simulink model "Asynchronous_motor"  (R2024a)
settings: Solver=VariableStepAuto  StartTime=0.0  StopTime=10.0  RelTol=1e-3
values from neighbouring files (symbols this model uses):
  B = 0    [setting.m]
  f_rated = 50    [setting.m]
  Ids_rated = V_max / sqrt(Rs^2 + (w_rated * Ls)^2)    [setting.m]
  J = 0.0252    [setting.m]
  Kac = 1 / Kpc    (= 0.063680128597)    [setting.m]
  Kas = 1 / Kps    [setting.m]
  Kic = R * wcc    (= 2896.1527295)    [setting.m]
  Kis = Kps * wcs / 5    [setting.m]
  Kpc = L * wcc    (= 15.7034858759)    [setting.m]
  Kps = J * wcs / Kt    [setting.m]
  Kt = 1.5 * np * Lm^2 * Ids_rated / Lr    [setting.m]
  Llr = 1.794e-3    (= 0.001794)    [setting.m]
  Lls = 1.794e-3    (= 0.001794)    [setting.m]
  np = 2    [setting.m]
  P_rated = 3700    [setting.m]
  pxyz = sqrt(3) *Tsw / Vdc    [setting.m]
  Rr = 0.379    [setting.m]
  Rs = 0.295    [setting.m]
  Te_rated = np * P_rated / (w_syn * (1 - s_rated))    (= 48.4005443375)    [setting.m]
  Tsw = 1 / fsw    (= 0.0001)    [setting.m]
  V_max = sqrt(2) / sqrt(3) * V_rated    [setting.m]
  V_rated = 220    [setting.m]
  Vdc = 500    [setting.m]
libraries: simulink x4, spsAsynchronousMachineSIUnitsLib x1, spsDCVoltageSourceLib x1, eeTransforms x1, spsUniversalBridgeLib x1, spsabctodq0Lib x1
settings Model: Creator=d  LastModifiedBy=d

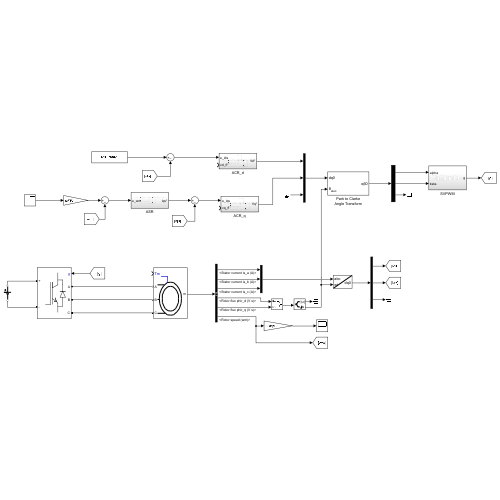
[thumbnail: Simulink's stored preview of the top-level diagram]
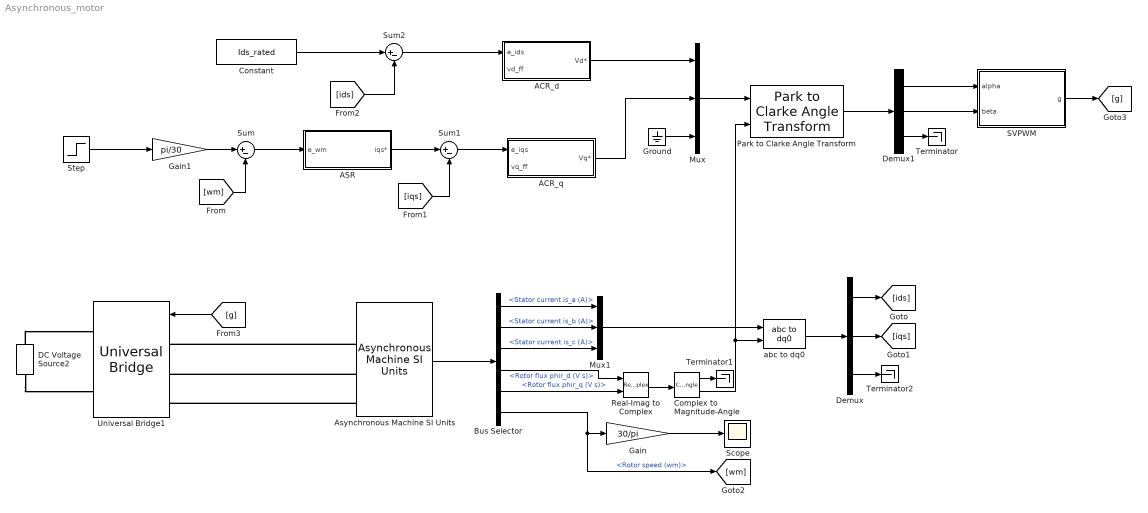
== system Asynchronous_motor ==
  ACR_d : Subsystem
  ACR_q : Subsystem
  ASR : Subsystem
  Asynchronous Machine SI Units : spsAsynchronousMachineSIUnitsLib/Asynchronous Machine SI Units  RotorType=Squirrel-cage  PresetModel=No  MechanicalLoad=Torque Tm  ShowDetailedParameters=on  ReferenceFrame=Stationary  Units=SI  MeasurementBus=off  NominalParameters=[P_rated V_rated f_rated]  VoltageRatio=1  Stator=[Rs Lls]  Rotor=[Rr Llr]  Cage1=[0.4155 0.002066]  Cage2=[0.4168 0.0003495]  Lm=Lm  Mechanical=[J B np]  PolePairs=2  InitialConditions=[1 0 0 0 0 0 0 0]  SimulateSaturation=off  Saturation=[14.03593122, 27.81365428, 53.79336849, 72.68890987, 97.98006896, 148.6815601, 215.7428561, 302.9841135, 428.7778367 ; 230, 322, 414, 460, 506, 552, 598, 644, 690]  LoadFlowParameters=1492000  TsPowergui=0  TsBlock=-1  IterativeModel=Trapezoidal non iterative  IterativeDiscreteModel=Trapezoidal non iterative  Pmec=1.492e+006
  Bus Selector : BusSelector  OutputSignals=Stator measurements.Stator current is_a (A),Stator measurements.Stator current is_b (A),Stator measurements.Stator current is_c (A),Rotor measurements.Rotor flux phir_d (V s),Rotor measurements.Rotor flux phir_q (V s),Mechanical.Rotor speed (wm)
  Complex to Magnitude-Angle : ComplexToMagnitudeAngle
  Constant : Constant  Value=Ids_rated
  DC Voltage Source2 : spsDCVoltageSourceLib/DC Voltage Source  Amplitude=Vdc  Measurements=None
  Demux : Demux  Outputs=3
  Demux1 : Demux  Outputs=3
  Gain : Gain  Gain=30/pi
  Gain1 : Gain  Gain=pi/30
  Ground : Ground
  Mux : Mux  Inputs=3
  Mux1 : Mux  Inputs=3
  Park to Clarke Angle Transform : eeTransforms/Park to Clarke Angle Transform  AxisAlignment=Q-axis
      settings: LibrarySourceBlock=|
      | ee_sl_lib/Mathematical
      | Transforms/Park to Clarke
      | Angle Transform
  Real-Imag to Complex : RealImagToComplex
  SVPWM : Subsystem
  Scope : Scope
  Step : Step  Time=0.4  Before=500  After=1400  SampleTime=0
  Sum : Sum  Inputs=|+-
  Sum1 : Sum  Inputs=|+-
  Sum2 : Sum  Inputs=|+-
  Terminator : Terminator
  Terminator1 : Terminator
  Terminator2 : Terminator
  Universal Bridge1 : spsUniversalBridgeLib/Universal Bridge  Arms=3  SnubberResistance=1e5  SnubberCapacitance=inf  Device=IGBT / Diodes  Ron=1e-3  Lon=0  ForwardVoltages="[  0  0  ]"  ForwardVoltage=0  GTOparameters=[ 10e-6 , 20e-6 ]  IGBTparameters=[ 1e-6 , 2e-6 ]  Measurements=None  Measurements_2=None  converterType=Rectifier
  abc to dq0 : spsabctodq0Lib/abc to dq0  Alignment=90 degrees behind phase A axis
  wires:
  Asynchronous Machine SI Units/1 -> Bus Selector/1
  Bus Selector/2 -> Mux1/2  "<Stator current is_b (A)>"
  Bus Selector/3 -> Mux1/3  "<Stator current is_c (A)>"
  Bus Selector/1 -> Mux1/1  "<Stator current is_a (A)>"
  Mux1/1 -> abc to dq0/1
  Complex to Magnitude-Angle/2 -> Park to Clarke Angle Transform/2, abc to dq0/2
  Bus Selector/5 -> Real-Imag to Complex/2  "<Rotor flux phir_q (V s)>"
  Bus Selector/6 -> [wm], Gain/1  "<Rotor speed (wm)>"
  Bus Selector/4 -> Real-Imag to Complex/1  "<Rotor flux phir_d (V s)>"
  Real-Imag to Complex/1 -> Complex to Magnitude-Angle/1
  Complex to Magnitude-Angle/1 -> Terminator1/1
  abc to dq0/1 -> Demux/1
  Demux/3 -> Terminator2/1
  Demux/1 -> [ids]
  Demux/2 -> [iqs]
  Gain/1 -> Scope/1
  Step/1 -> Gain1/1
  Gain1/1 -> Sum/1
  [wm] -> Sum/2
  Sum/1 -> ASR/1(e_wm)
  ASR/1(iqs*) -> Sum1/1
  [iqs] -> Sum1/2
  Sum1/1 -> ACR_q/1(e_iqs)
  Constant/1 -> Sum2/1
  [ids] -> Sum2/2
  Sum2/1 -> ACR_d/1(e_ids)
  ACR_d/1(Vd*) -> Mux/1
  ACR_q/1(Vq*) -> Mux/2
  Mux/1 -> Park to Clarke Angle Transform/1
  Ground/1 -> Mux/3
  Park to Clarke Angle Transform/1 -> Demux1/1
  Demux1/3 -> Terminator/1
  Demux1/1 -> SVPWM/1(alpha)
  Demux1/2 -> SVPWM/2(beta)
  SVPWM/1(g) -> [g]
  [g] -> Universal Bridge1/1
  connections:
  DC Voltage Source2/RConn1 -- Universal Bridge1/RConn1
  DC Voltage Source2/LConn1 -- Universal Bridge1/RConn2
  Asynchronous Machine SI Units/LConn1 -- Universal Bridge1/LConn1
  Asynchronous Machine SI Units/LConn2 -- Universal Bridge1/LConn2
  Asynchronous Machine SI Units/LConn3 -- Universal Bridge1/LConn3

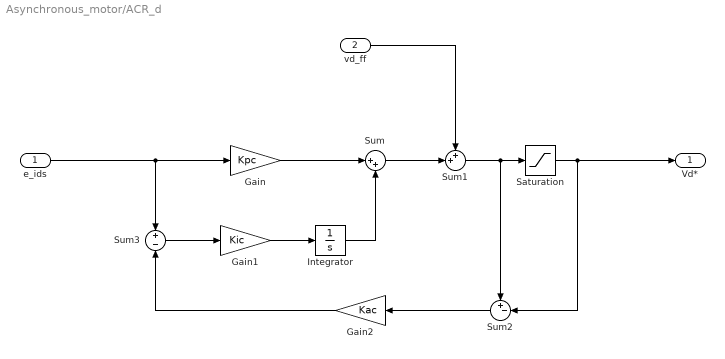
== system Asynchronous_motor/ACR_d ==
  e_ids : Inport
  vd_ff : Inport  Port=2
  Gain : Gain  Gain=Kpc
  Gain1 : Gain  Gain=Kic
  Gain2 : Gain  Gain=Kac
  Integrator : Integrator
  Saturation : Saturate  UpperLimit=V_max * 2  LowerLimit=-V_max * 2
  Sum : Sum  Inputs=|++
  Sum1 : Sum  Inputs=++|
  Sum2 : Sum  Inputs=+-|
  Sum3 : Sum  Inputs=+|-
  Vd* : Outport
  wires:
  e_ids/1 -> Sum3/1, Gain/1
  Gain1/1 -> Integrator/1
  Gain/1 -> Sum/1
  Integrator/1 -> Sum/2
  Sum/1 -> Sum1/2
  vd_ff/1 -> Sum1/1
  Sum1/1 -> Saturation/1, Sum2/1
  Saturation/1 -> Sum2/2, Vd*/1
  Sum2/1 -> Gain2/1
  Sum3/1 -> Gain1/1
  Gain2/1 -> Sum3/2

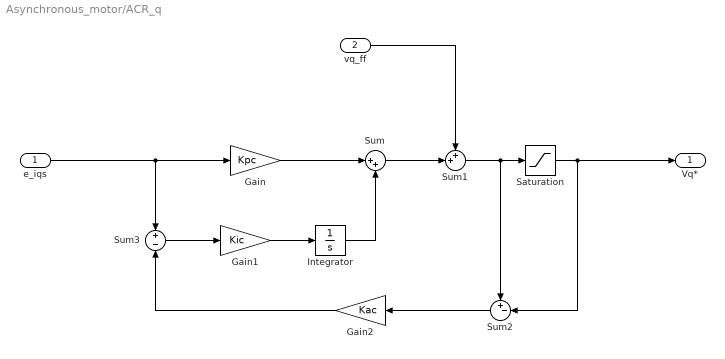
== system Asynchronous_motor/ACR_q ==
  e_iqs : Inport
  vq_ff : Inport  Port=2
  Gain : Gain  Gain=Kpc
  Gain1 : Gain  Gain=Kic
  Gain2 : Gain  Gain=Kac
  Integrator : Integrator
  Saturation : Saturate  UpperLimit=V_max * 2  LowerLimit=-V_max * 2
  Sum : Sum  Inputs=|++
  Sum1 : Sum  Inputs=++|
  Sum2 : Sum  Inputs=+-|
  Sum3 : Sum  Inputs=+|-
  Vq* : Outport
  wires:
  e_iqs/1 -> Sum3/1, Gain/1
  Gain1/1 -> Integrator/1
  Gain/1 -> Sum/1
  Integrator/1 -> Sum/2
  Sum/1 -> Sum1/2
  vq_ff/1 -> Sum1/1
  Sum1/1 -> Saturation/1, Sum2/1
  Saturation/1 -> Sum2/2, Vq*/1
  Sum2/1 -> Gain2/1
  Sum3/1 -> Gain1/1
  Gain2/1 -> Sum3/2

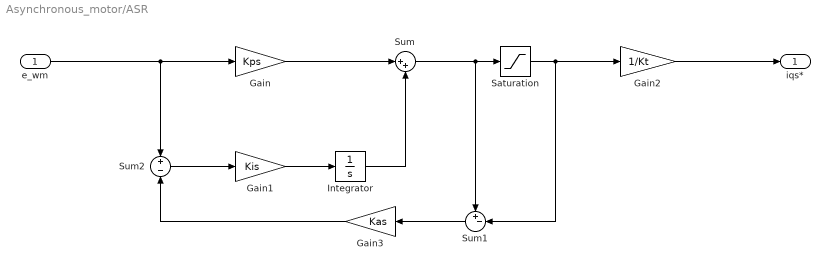
== system Asynchronous_motor/ASR ==
  e_wm : Inport
  Gain : Gain  Gain=Kps
  Gain1 : Gain  Gain=Kis
  Gain2 : Gain  Gain=1/Kt
  Gain3 : Gain  Gain=Kas
  Integrator : Integrator
  Saturation : Saturate  UpperLimit=Te_rated  LowerLimit=-Te_rated
  Sum : Sum  Inputs=|++
  Sum1 : Sum  Inputs=+-|
  Sum2 : Sum  Inputs=+|-
  iqs* : Outport
  wires:
  e_wm/1 -> Sum2/1, Gain/1
  Gain1/1 -> Integrator/1
  Gain/1 -> Sum/1
  Integrator/1 -> Sum/2
  Sum/1 -> Sum1/1, Saturation/1
  Saturation/1 -> Sum1/2, Gain2/1
  Gain2/1 -> iqs*/1
  Sum1/1 -> Gain3/1
  Sum2/1 -> Gain1/1
  Gain3/1 -> Sum2/2

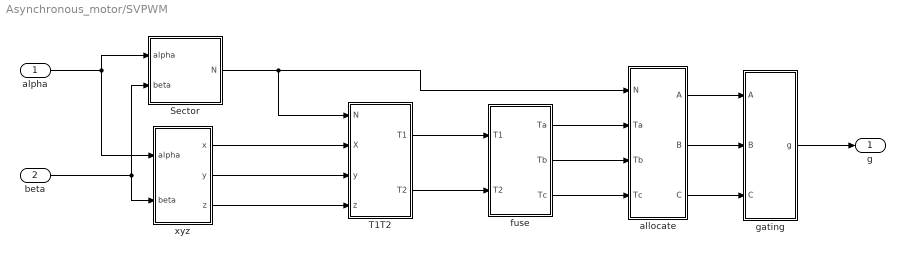
== system Asynchronous_motor/SVPWM ==
  alpha : Inport
  beta : Inport  Port=2
  Sector : Subsystem
  T1T2 : Subsystem
  allocate : Subsystem
  fuse : Subsystem
  gating : Subsystem
  xyz : Subsystem
  g : Outport
  wires:
  allocate/3(C) -> gating/3(C)
  fuse/2(Tb) -> allocate/3(Tb)
  allocate/1(A) -> gating/1(A)
  allocate/2(B) -> gating/2(B)
  xyz/2(y) -> T1T2/3(y)
  T1T2/1(T1) -> fuse/1(T1)
  xyz/3(z) -> T1T2/4(z)
  T1T2/2(T2) -> fuse/2(T2)
  fuse/3(Tc) -> allocate/4(Tc)
  Sector/1(N) -> T1T2/1(N), allocate/1(N)
  fuse/1(Ta) -> allocate/2(Ta)
  xyz/1(x) -> T1T2/2(X)
  alpha/1 -> Sector/1(alpha), xyz/1(alpha)
  beta/1 -> Sector/2(beta), xyz/2(beta)
  gating/1(g) -> g/1

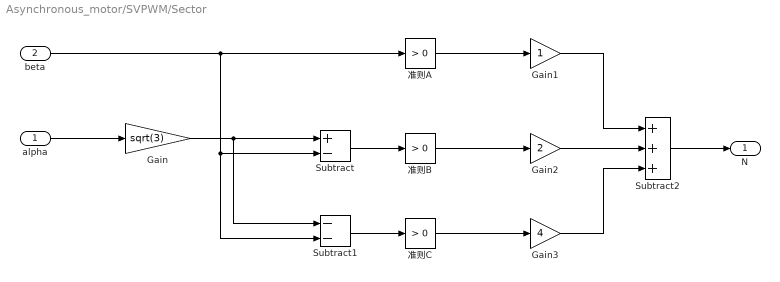
== system Asynchronous_motor/SVPWM/Sector ==
  alpha : Inport
  beta : Inport  Port=2
  Gain : Gain  Gain=sqrt(3)
  Gain1 : Gain
  Gain2 : Gain  Gain=2
  Gain3 : Gain  Gain=4
  Subtract : Sum  Inputs=+-
  Subtract1 : Sum  Inputs=--
  Subtract2 : Sum  Inputs=+++
  准则A : simulink/Logic and Bit Operations/Compare To Constant  relop=>  const=0  OutDataTypeStr=boolean
  准则B : simulink/Logic and Bit Operations/Compare To Constant  relop=>  const=0  OutDataTypeStr=boolean
  准则C : simulink/Logic and Bit Operations/Compare To Constant  relop=>  const=0  OutDataTypeStr=boolean
  N : Outport
  wires:
  beta/1 -> Subtract1/2, Subtract/2, 准则A/1
  alpha/1 -> Gain/1
  Gain/1 -> Subtract1/1, Subtract/1
  Subtract/1 -> 准则B/1
  Subtract1/1 -> 准则C/1
  准则C/1 -> Gain3/1
  准则B/1 -> Gain2/1
  准则A/1 -> Gain1/1
  Gain1/1 -> Subtract2/1
  Gain2/1 -> Subtract2/2
  Gain3/1 -> Subtract2/3
  Subtract2/1 -> N/1

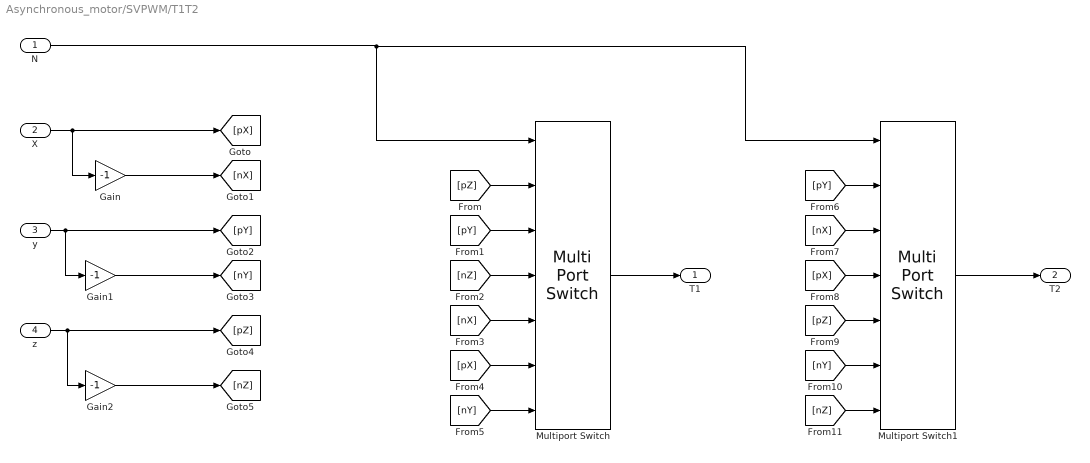
== system Asynchronous_motor/SVPWM/T1T2 ==
  N : Inport
  X : Inport  Port=2
  y : Inport  Port=3
  z : Inport  Port=4
  Gain : Gain  Gain=-1
  Gain1 : Gain  Gain=-1
  Gain2 : Gain  Gain=-1
  Multiport Switch : MultiPortSwitch  Inputs=6  SaturateOnIntegerOverflow=off  InputSameDT=off
  Multiport Switch1 : MultiPortSwitch  Inputs=6  SaturateOnIntegerOverflow=off  InputSameDT=off
  T1 : Outport
  T2 : Outport  Port=2
  wires:
  X/1 -> [pX], Gain/1
  y/1 -> [pY], Gain1/1
  z/1 -> Gain2/1, [pZ]
  Gain/1 -> [nX]
  Gain1/1 -> [nY]
  Gain2/1 -> [nZ]
  Multiport Switch/1 -> T1/1
  Multiport Switch1/1 -> T2/1
  N/1 -> Multiport Switch1/1, Multiport Switch/1
  [pZ] -> Multiport Switch/2
  [pY] -> Multiport Switch/3
  [nZ] -> Multiport Switch/4
  [nX] -> Multiport Switch/5
  [pX] -> Multiport Switch/6
  [nY] -> Multiport Switch/7
  [pY] -> Multiport Switch1/2
  [nX] -> Multiport Switch1/3
  [pX] -> Multiport Switch1/4
  [pZ] -> Multiport Switch1/5
  [nY] -> Multiport Switch1/6
  [nZ] -> Multiport Switch1/7

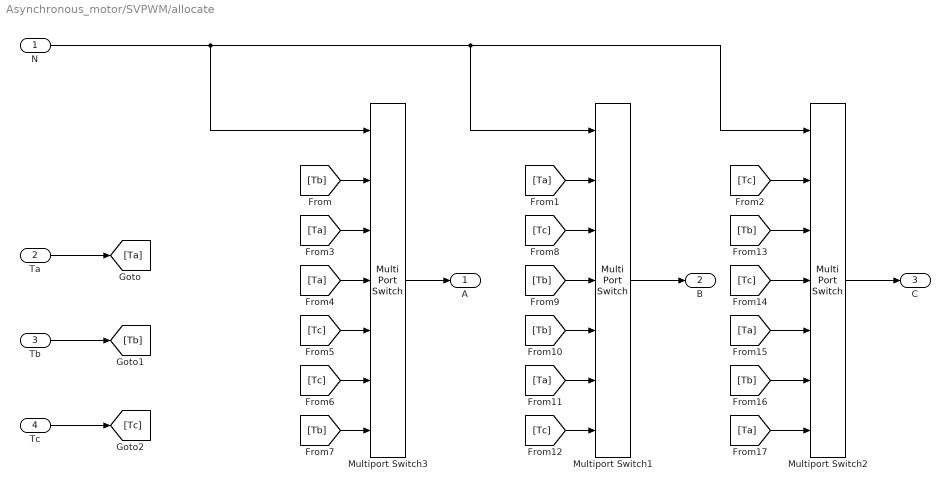
== system Asynchronous_motor/SVPWM/allocate ==
  N : Inport
  Ta : Inport  Port=2
  Tb : Inport  Port=3
  Tc : Inport  Port=4
  Multiport Switch1 : MultiPortSwitch  Inputs=6  SaturateOnIntegerOverflow=off  InputSameDT=off
  Multiport Switch2 : MultiPortSwitch  Inputs=6  SaturateOnIntegerOverflow=off  InputSameDT=off
  Multiport Switch3 : MultiPortSwitch  Inputs=6  SaturateOnIntegerOverflow=off  InputSameDT=off
  A : Outport
  B : Outport  Port=2
  C : Outport  Port=3
  wires:
  Tc/1 -> [Tc]
  Tb/1 -> [Tb]
  Ta/1 -> [Ta]
  Multiport Switch2/1 -> C/1
  Multiport Switch3/1 -> A/1
  Multiport Switch1/1 -> B/1
  N/1 -> Multiport Switch3/1, Multiport Switch1/1, Multiport Switch2/1
  [Tb] -> Multiport Switch3/2
  [Ta] -> Multiport Switch1/2
  [Tc] -> Multiport Switch2/2
  [Ta] -> Multiport Switch3/3
  [Ta] -> Multiport Switch3/4
  [Tc] -> Multiport Switch3/5
  [Tc] -> Multiport Switch3/6
  [Tb] -> Multiport Switch3/7
  [Tc] -> Multiport Switch1/3
  [Tb] -> Multiport Switch1/4
  [Tb] -> Multiport Switch1/5
  [Ta] -> Multiport Switch1/6
  [Tc] -> Multiport Switch1/7
  [Tb] -> Multiport Switch2/3
  [Tc] -> Multiport Switch2/4
  [Ta] -> Multiport Switch2/5
  [Tb] -> Multiport Switch2/6
  [Ta] -> Multiport Switch2/7

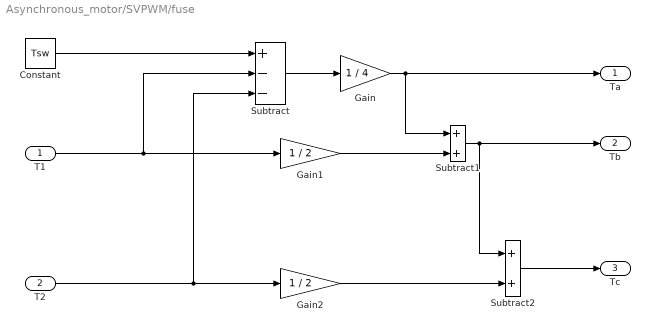
== system Asynchronous_motor/SVPWM/fuse ==
  T1 : Inport
  T2 : Inport  Port=2
  Constant : Constant  Value=Tsw
  Gain : Gain  Gain=1 / 4
  Gain1 : Gain  Gain=1 / 2
  Gain2 : Gain  Gain=1 / 2
  Subtract : Sum  Inputs=+--
  Subtract1 : Sum
  Subtract2 : Sum
  Ta : Outport
  Tb : Outport  Port=2
  Tc : Outport  Port=3
  wires:
  Constant/1 -> Subtract/1
  T1/1 -> Gain1/1, Subtract/2
  T2/1 -> Gain2/1, Subtract/3
  Subtract/1 -> Gain/1
  Gain/1 -> Subtract1/1, Ta/1
  Gain1/1 -> Subtract1/2
  Subtract1/1 -> Subtract2/1, Tb/1
  Subtract2/1 -> Tc/1
  Gain2/1 -> Subtract2/2

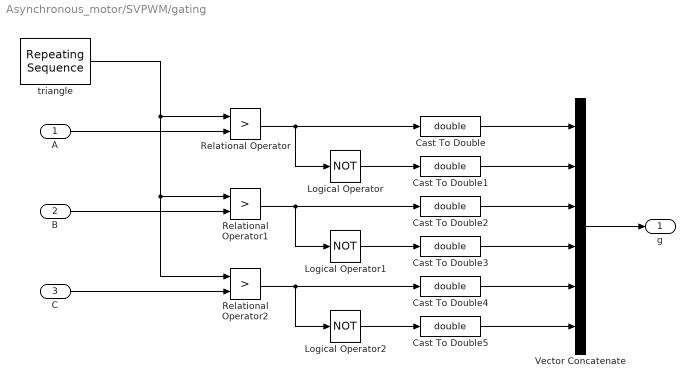
== system Asynchronous_motor/SVPWM/gating ==
  A : Inport
  B : Inport  Port=2
  C : Inport  Port=3
  Cast To Double{,1..5} (6 alike) : DataTypeConversion  OutDataTypeStr=double  SaturateOnIntegerOverflow=off  RndMeth=Floor
  Logical Operator : Logic  Operator=NOT  AllPortsSameDT=off  OutDataTypeStr=boolean
  Logical Operator1 : Logic  Operator=NOT  AllPortsSameDT=off  OutDataTypeStr=boolean
  Logical Operator2 : Logic  Operator=NOT  AllPortsSameDT=off  OutDataTypeStr=boolean
  Relational Operator : RelationalOperator  Operator=>  OutDataTypeStr=boolean  RndMeth=Simplest  InputSameDT=off
  Relational Operator1 : RelationalOperator  Operator=>  OutDataTypeStr=boolean  RndMeth=Simplest  InputSameDT=off
  Relational Operator2 : RelationalOperator  Operator=>  OutDataTypeStr=boolean  RndMeth=Simplest  InputSameDT=off
  Vector Concatenate : Concatenate  NumInputs=6
  triangle : simulink/Sources/Repeating Sequence  rep_seq_t=[0 Tsw/2 Tsw]  rep_seq_y=[0 Tsw/2 0]
  g : Outport
  wires:
  triangle/1 -> Relational Operator/1, Relational Operator2/1, Relational Operator1/1
  A/1 -> Relational Operator/2
  B/1 -> Relational Operator1/2
  C/1 -> Relational Operator2/2
  Relational Operator1/1 -> Cast To Double2/1, Logical Operator1/1
  Relational Operator/1 -> Cast To Double/1, Logical Operator/1
  Relational Operator2/1 -> Cast To Double4/1, Logical Operator2/1
  Logical Operator/1 -> Cast To Double1/1
  Logical Operator1/1 -> Cast To Double3/1
  Logical Operator2/1 -> Cast To Double5/1
  Cast To Double/1 -> Vector Concatenate/1
  Cast To Double1/1 -> Vector Concatenate/2
  Cast To Double2/1 -> Vector Concatenate/3
  Cast To Double3/1 -> Vector Concatenate/4
  Cast To Double4/1 -> Vector Concatenate/5
  Cast To Double5/1 -> Vector Concatenate/6
  Vector Concatenate/1 -> g/1

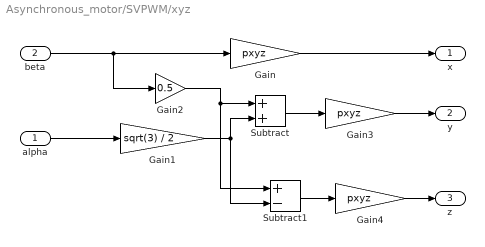
== system Asynchronous_motor/SVPWM/xyz ==
  alpha : Inport
  beta : Inport  Port=2
  Gain : Gain  Gain=pxyz
  Gain1 : Gain  Gain=sqrt(3) / 2
  Gain2 : Gain  Gain=0.5
  Gain3 : Gain  Gain=pxyz
  Gain4 : Gain  Gain=pxyz
  Subtract : Sum
  Subtract1 : Sum  Inputs=+-
  x : Outport
  y : Outport  Port=2
  z : Outport  Port=3
  wires:
  beta/1 -> Gain2/1, Gain/1
  Gain/1 -> x/1
  alpha/1 -> Gain1/1
  Gain2/1 -> Subtract1/1, Subtract/1
  Gain1/1 -> Subtract/2, Subtract1/2
  Gain3/1 -> y/1
  Subtract/1 -> Gain3/1
  Gain4/1 -> z/1
  Subtract1/1 -> Gain4/1
